simulink model "parte4_eje1_Thidraulica_mdl"  (R2017b)
settings: Solver=VariableStepAuto  StartTime=0.0  StopTime=20  RelTol=1e-3
libraries: simulink x2
settings Model: Creator=cjuar  LastModifiedBy=Admon

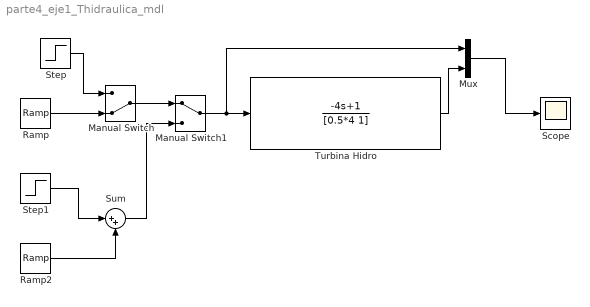
== system parte4_eje1_Thidraulica_mdl ==
  Manual Switch : ManualSwitch  CurrentSetting=0
  Manual Switch1 : ManualSwitch
  Mux : Mux  Inputs=2
  Ramp : simulink/Sources/Ramp  slope=1  start=0  X0=0
  Ramp2 : simulink/Sources/Ramp  slope=-1  start=10  X0=0
  Scope : Scope
  Step : Step  SampleTime=0
  Step1 : Step  SampleTime=0
  Sum : Sum  Inputs=|++
  Turbina Hidro : TransferFcn  Numerator=[-4 1]  Denominator=[0.5*4 1]
  wires:
  Step/1 -> Manual Switch/1
  Ramp/1 -> Manual Switch/2
  Manual Switch/1 -> Manual Switch1/1
  Step1/1 -> Sum/1
  Ramp2/1 -> Sum/2
  Sum/1 -> Manual Switch1/2
  Turbina Hidro/1 -> Mux/2
  Mux/1 -> Scope/1
  Manual Switch1/1 -> Mux/1, Turbina Hidro/1
